simulink model "gm_HDLHeaderScrambler_vs"  (R2024a)
settings: Solver=FixedStepDiscrete  StartTime=0.0  StopTime=stopTime  RelTol=1e-3
values from neighbouring files (symbols this model uses):
  fs = 1    [testHeaderScrambler.m]
undefined symbols (not defined in the file or in its folder): clk, clk_enable, reset_x
libraries: hdlsllib x23, simulink x4, dspsrcs4 x2, whdlutilities x1, vivadosimlib x1, HDL_ieee_8021513 x1
settings Model: Creator=cotti  LastModifiedBy=cotti
settings OptimizationCC: BlockReduction=off  ConditionallyExecuteInputs=off  DefaultParameterBehavior=Inlined  InheritOutputTypeSmallerThanSingle=on
settings DebuggingCC: AlgebraicLoopMsg=error  ArtificialAlgebraicLoopMsg=error  InheritedTsInSrcMsg=none  SingleTaskRateTransMsg=error  UnconnectedInputMsg=warning  UnconnectedOutputMsg=warning  UnconnectedLineMsg=warning
settings HardwareCC: ProdBitPerPointer=32  ProdBitPerSizeT=32  ProdBitPerPtrDiffT=32  ProdLargestAtomicFloat=None  ProdIntDivRoundTo=Undefined  ProdEndianess=Unspecified  ProdWordSize=32  ProdHWDeviceType=ASIC/FPGA->ASIC/FPGA  TargetBitPerLong=64  TargetBitPerPointer=64  TargetBitPerSizeT=64  TargetBitPerPtrDiffT=64  TargetLongLongMode=on  TargetIntDivRoundTo=Zero  TargetEndianess=LittleEndian  TargetWordSize=64  TargetHWDeviceType=Custom Processor->MATLAB Host Computer  ProdEqTarget=off

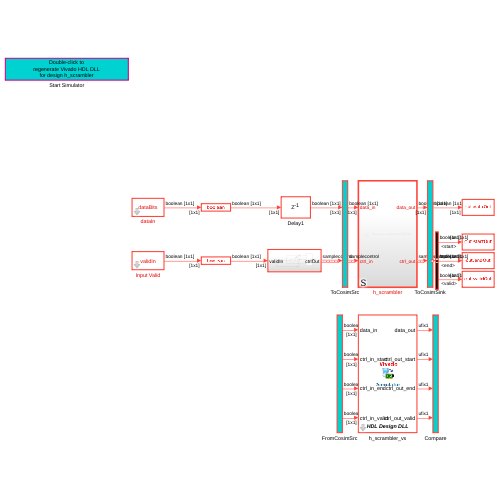
[thumbnail: Simulink's stored preview of the top-level diagram]
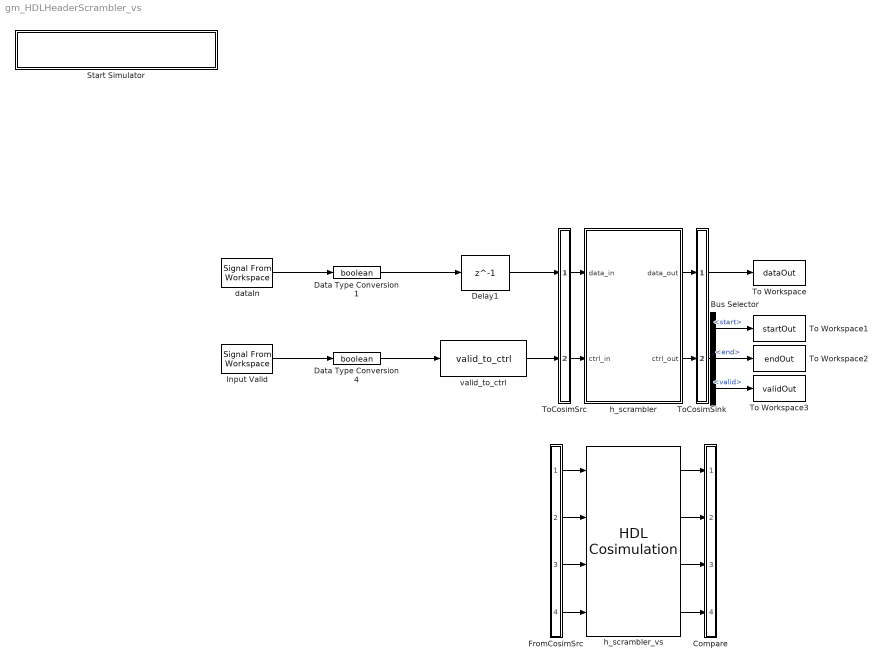
== system gm_HDLHeaderScrambler_vs ==
  Bus Selector : BusSelector  OutputSignals=start,end,valid
  Compare : Subsystem
      mask Display: disp('')
  Data Type Conversion1 : DataTypeConversion  OutDataTypeStr=boolean  SaturateOnIntegerOverflow=off  RndMeth=Floor
  Data Type Conversion4 : DataTypeConversion  OutDataTypeStr=boolean  SaturateOnIntegerOverflow=off  RndMeth=Floor
  Delay1 : Delay  DelayLength=1  InitialCondition=0  UseCircularBuffer=on
  FromCosimSrc : Subsystem
      mask Display: disp('')
  Input Valid : dspsrcs4/Signal From Workspace  X=validIn  Ts=1/fs  nsamps=1  OutputAfterFinalValue=Setting to zero  ignoreOrWarnInputAndFrameLengths=off  OutputFrames=off
  Start Simulator : Subsystem
      settings: OpenFcn=|
      | cosimDirName = pwd;
      | cd 'hdl_prj/hdlsrc/HDLHeaderScrambler';
      | [s,r] = system('vivado -mode batch -source gm_HDLHeaderScrambler_vs.tcl','-echo');
      | cd (cosimDirName);
      | clear cosimDirName;
      | if s
      |    error('Failed to create Vivado HDL design DLL using script gm_HDLHeaderScrambler_vs.tcl.');
      | end
      mask Display: disp('Double-click to\nregenerate Vivado HDL DLL\nfor design h_scrambler')
  To Workspace : ToWorkspace  VariableName=dataOut  SampleTime=1/fs
      settings: Save2DSignal=2-D array (concatenate along first dimension)
  To Workspace1 : ToWorkspace  VariableName=startOut  SampleTime=1/fs
      settings: Save2DSignal=2-D array (concatenate along first dimension)
  To Workspace2 : ToWorkspace  VariableName=endOut  SampleTime=1/fs
      settings: Save2DSignal=2-D array (concatenate along first dimension)
  To Workspace3 : ToWorkspace  VariableName=validOut  SampleTime=1/fs
      settings: Save2DSignal=2-D array (concatenate along first dimension)
  ToCosimSink : Subsystem
      mask Display: disp('')
  ToCosimSrc : Subsystem
      mask Display: disp('')
  dataIn : dspsrcs4/Signal From Workspace  X=dataBits  Ts=1/fs  nsamps=1  OutputAfterFinalValue=Setting to zero  ignoreOrWarnInputAndFrameLengths=off  OutputFrames=off
  h_scrambler : Subsystem
      settings: LibrarySourceBlock=|
      | hdlsllib/Ports &
      | Subsystems/Subsystem
  h_scrambler_vs : vivadosimlib/HDL Cosimulation  PortPaths=/h_scrambler/data_in;/h_scrambler/ctrl_in_start;/h_scrambler/ctrl_in_end;/h_scrambler/ctrl_in_valid;/h_scrambler/data_out;/h_scrambler/ctrl_out_start;/h_scrambler/ctrl_out_end;/h_scrambler/ctrl_out_valid  PortModes=[1 1 1 1 2 2 2 2 ]  PortTimes=[-1 -1 -1 -1 1 1 1 1 ]  PortSigns=[-1 -1 -1 -1 0 0 0 0 ]  PortFracLengths=[0,0,0,0,0,0,0,0]  PortWordLengths=[-1,-1,-1,-1,1,1,1,1]  PortHDLWordSizes=[1,1,1,1,1,1,1,1]  CommLocal=on  CommSharedMemory=on  CommPortNumber=4449  CommShowInfo=on  ClockPaths=clk;clk_enable;reset_x;  ClockModes=[2 4 3]  ClockTimes=[1e-08 3.7e-08 2.7e-08]  TclPostSimCommand="puts \"done\""  TimingMode=ns  TimingScaleFactor=10  idxCellArray={'UNUSED_VAR'}  CosimBypass=Full Simulation  AllowDirectFeedthrough=on  ProductName=EDA Simulator Link VS  RunAutoTimescale=off  HdlClocks=0  PreRunTime=40  PreRunTimeUnit=ns
  valid_to_ctrl : HDL_ieee_8021513/valid_to_ctrl  SystemSampleTime=-1  VariantActivationTime=update diagram  AllowFlexibleInterface=on  Latency=0  AutoFrameSizeCalculation=off
      settings: SourceProductName=HDL IEEE 8021513
  wires:
  Bus Selector/2 -> To Workspace2/1  "<end>"
  Bus Selector/3 -> To Workspace3/1  "<valid>"
  Bus Selector/1 -> To Workspace1/1  "<start>"
  Data Type Conversion1/1 -> Delay1/1
  dataIn/1 -> Data Type Conversion1/1
  Data Type Conversion4/1 -> valid_to_ctrl/1
  Input Valid/1 -> Data Type Conversion4/1
  ToCosimSrc/1(out1) -> h_scrambler/1(data_in)
  ToCosimSrc/2(out2) -> h_scrambler/2(ctrl_in)
  h_scrambler/1(data_out) -> ToCosimSink/1(in1)
  h_scrambler/2(ctrl_out) -> ToCosimSink/2(in2)
  Delay1/1 -> ToCosimSrc/1(in1)
  valid_to_ctrl/1 -> ToCosimSrc/2(in2)
  ToCosimSink/1(out1) -> To Workspace/1
  ToCosimSink/2(out2) -> Bus Selector/1
  FromCosimSrc/1(out1) -> h_scrambler_vs/1
  FromCosimSrc/2(out2) -> h_scrambler_vs/2
  FromCosimSrc/3(out3) -> h_scrambler_vs/3
  FromCosimSrc/4(out4) -> h_scrambler_vs/4
  h_scrambler_vs/1 -> Compare/1(in1)
  h_scrambler_vs/2 -> Compare/2(in2)
  h_scrambler_vs/3 -> Compare/3(in3)
  h_scrambler_vs/4 -> Compare/4(in4)

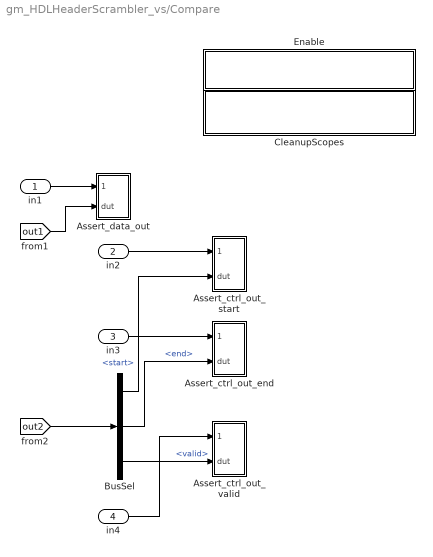
== system gm_HDLHeaderScrambler_vs/Compare ==
  in1 : Inport
  in2 : Inport  Port=2
  in3 : Inport  Port=3
  in4 : Inport  Port=4
  Assert_ctrl_out_end : Subsystem
      settings: LibrarySourceBlock=hdlmdlgenlib/AssertEq
  Assert_ctrl_out_start : Subsystem
      settings: LibrarySourceBlock=hdlmdlgenlib/AssertEq
  Assert_ctrl_out_valid : Subsystem
      settings: LibrarySourceBlock=hdlmdlgenlib/AssertEq
  Assert_data_out : Subsystem
      settings: LibrarySourceBlock=hdlmdlgenlib/AssertEq
  BusSel : BusSelector  OutputSignals=start,end,valid
  CleanupScopes : Subsystem
      settings: OpenFcn=|
      | blkName = gcb; %self block
      | idx = regexp(blkName, '/CleanupScopes$', 'once');
      | blkParent = blkName(1:idx-1);
      | blks=find_system(blkParent, 'LookUnderMasks', 'all','blocktype', 'Scope');
      | for itr = 1:length(blks)
      | 	 hScopeCfg = get_param(blks{itr},'ScopeConfiguration');
      | 	 hScopeCfg.Visible = ~ hScopeCfg.Visible;
      | end
      | drawnow;
      mask Display: fprintf(message('hdlcoder:cosim:vnl_dblclick').getString());
  Enable : Subsystem
      settings: OpenFcn=|
      | blkName = gcb;
      | idx = regexp(blkName, '/Enable$', 'once');
      | blkParent = blkName(1:idx-1);
      | blks=find_system(blkParent, 'LookUnderMasks', 'all','blocktype', 'Assertion');
      | e = get_param(blks{1}, 'Enabled');
      | if strcmp(e, 'on'), f= 'off';, else, f = 'on';, end
      | for ii=1:length(blks), set_param(blks{ii}, 'Enabled', f);, end
      | set_param(gcb, 'MaskDisplay',['fprintf(message(''hdlcoder:cosim:vnl_dblclick_assertions'',','''',upper(e),'''',').getString())']);
      mask Display: fprintf(message('hdlcoder:cosim:vnl_dblclick_assertions','OFF').getString());
  wires:
  BusSel/1 -> Assert_ctrl_out_start/2(dut)  "<start>"
  BusSel/3 -> Assert_ctrl_out_valid/2(dut)  "<valid>"
  BusSel/2 -> Assert_ctrl_out_end/2(dut)  "<end>"
  in3/1 -> Assert_ctrl_out_end/1(cosim)
  in2/1 -> Assert_ctrl_out_start/1(cosim)
  in4/1 -> Assert_ctrl_out_valid/1(cosim)
  [out2] -> BusSel/1
  [out1] -> Assert_data_out/2(dut)
  in1/1 -> Assert_data_out/1(cosim)

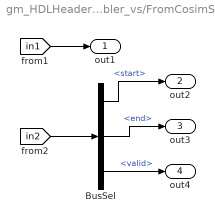
== system gm_HDLHeaderScrambler_vs/FromCosimSrc ==
  BusSel : BusSelector  OutputSignals=start,end,valid
  out1 : Outport
  out2 : Outport  Port=2
  out3 : Outport  Port=3
  out4 : Outport  Port=4
  wires:
  BusSel/3 -> out4/1  "<valid>"
  BusSel/2 -> out3/1  "<end>"
  BusSel/1 -> out2/1  "<start>"
  [in2] -> BusSel/1
  [in1] -> out1/1

== system gm_HDLHeaderScrambler_vs/Start Simulator ==

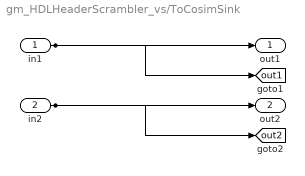
== system gm_HDLHeaderScrambler_vs/ToCosimSink ==
  in1 : Inport
  in2 : Inport  Port=2
  out1 : Outport
  out2 : Outport  Port=2
  tag scope: out1=global, out2=global
  wires:
  in1/1 -> out1/1, [out1]
  in2/1 -> out2/1, [out2]

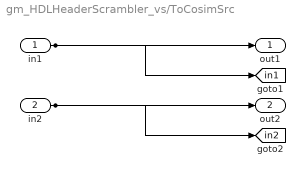
== system gm_HDLHeaderScrambler_vs/ToCosimSrc ==
  in1 : Inport
  in2 : Inport  Port=2
  out1 : Outport
  out2 : Outport  Port=2
  tag scope: in1=global, in2=global
  wires:
  in1/1 -> out1/1, [in1]
  in2/1 -> out2/1, [in2]

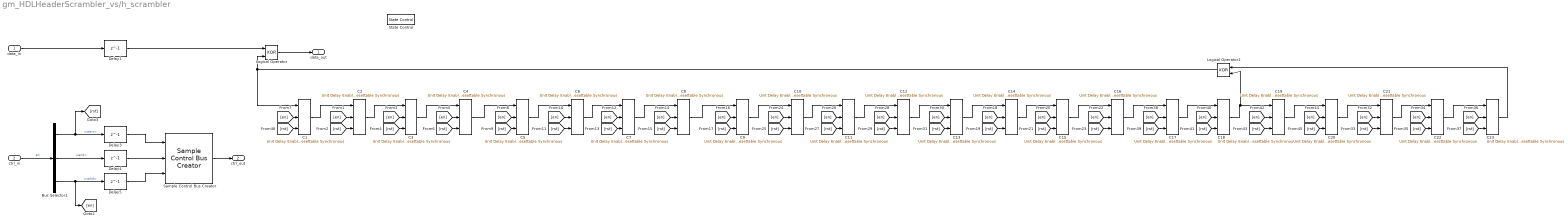
== system gm_HDLHeaderScrambler_vs/h_scrambler ==
  data_in : Inport
  ctrl_in : Inport  Port=2
  Bus Selector1 : BusSelector  OutputSignals=start,end,valid
  C{1,3,5,7,9,11,13,15,17,19,21,23} (12 alike) : hdlsllib/Discrete/Unit Delay Enabled Resettable Synchronous  InitialCondition=0  SampleTime=-1
  C{2,4,6,8,10,12,14,16,18,20,22} (11 alike) : hdlsllib/Discrete/Unit Delay Enabled Resettable Synchronous  InitialCondition=1  SampleTime=-1
  Delay{1,3..5} (4 alike) : Delay  DelayLength=1  InitialCondition=0  UseCircularBuffer=on
  Logical Operator : Logic  Operator=XOR  IconShape=distinctive  AllPortsSameDT=off  OutDataTypeStr=boolean
  Logical Operator1 : Logic  Operator=XOR  IconShape=distinctive  AllPortsSameDT=off  OutDataTypeStr=boolean
  Sample Control Bus Creator : whdlutilities/Sample Control Bus Creator
  State Control : StateControl  StateControl=Synchronous
  data_out : Outport
  ctrl_out : Outport  Port=2  VectorParamsAs1DForOutWhenUnconnected=off
  wires:
  Sample Control Bus Creator/1 -> ctrl_out/1
  Delay5/1 -> Sample Control Bus Creator/3
  Delay4/1 -> Sample Control Bus Creator/2
  Delay3/1 -> Sample Control Bus Creator/1
  Bus Selector1/3 -> Delay5/1, [en]  "<valid>"
  Bus Selector1/2 -> Delay4/1  "<end>"
  Bus Selector1/1 -> Delay3/1, [rst]  "<start>"
  C23/1 -> Logical Operator1/1
  [rst] -> C22/3
  C19/1 -> C20/1
  [en] -> C20/2
  [en] -> C21/2
  C21/1 -> C22/1
  [rst] -> C18/3
  [en] -> C17/2
  [rst] -> C19/3
  [rst] -> C21/3
  C17/1 -> C18/1
  C22/1 -> C23/1
  [en] -> C19/2
  [en] -> C18/2
  [en] -> C23/2
  [rst] -> C20/3
  [en] -> C22/2
  C16/1 -> C17/1
  [rst] -> C23/3
  [rst] -> C17/3
  C8/1 -> C9/1
  [rst] -> C15/3
  [en] -> C15/2
  [en] -> C14/2
  [rst] -> C16/3
  [en] -> C12/2
  [rst] -> C14/3
  C13/1 -> C14/1
  C11/1 -> C12/1
  [rst] -> C9/3
  [en] -> C10/2
  [en] -> C9/2
  C14/1 -> C15/1
  [en] -> C11/2
  [rst] -> C13/3
  C10/1 -> C11/1
  [rst] -> C10/3
  C12/1 -> C13/1
  [en] -> C13/2
  [rst] -> C11/3
  [en] -> C16/2
  [rst] -> C12/3
  C9/1 -> C10/1
  C15/1 -> C16/1
  [rst] -> C5/3
  [en] -> C6/2
  C6/1 -> C7/1
  [en] -> C8/2
  [rst] -> C6/3
  C5/1 -> C6/1
  [rst] -> C7/3
  C7/1 -> C8/1
  [rst] -> C8/3
  [en] -> C7/2
  [en] -> C5/2
  Delay1/1 -> Logical Operator/1
  data_in/1 -> Delay1/1
  ctrl_in/1 -> Bus Selector1/1  "en"
  Logical Operator/1 -> data_out/1
  [rst] -> C3/3
  [en] -> C3/2
  Logical Operator1/1 -> Logical Operator/2, C1/1
  [rst] -> C2/3
  C1/1 -> C2/1
  C3/1 -> C4/1
  [en] -> C1/2
  [rst] -> C1/3
  C4/1 -> C5/1
  [en] -> C4/2
  C2/1 -> C3/1
  [rst] -> C4/3
  [en] -> C2/2
  C20/1 -> C21/1
  C18/1 -> Logical Operator1/2, C19/1

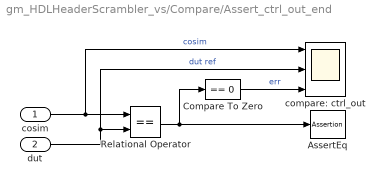
== system gm_HDLHeaderScrambler_vs/Compare/Assert_ctrl_out_end ==
  cosim : Inport
  dut : Inport  Port=2
  AssertEq : Assertion
  Compare To Zero : simulink/Logic and Bit Operations/Compare To Zero  relop===  OutDataTypeStr=boolean
  Relational Operator : RelationalOperator  Operator===  OutDataTypeStr=boolean  InputSameDT=off
  compare: ctrl_out : Scope  NumInputPorts=3
  wires:
  Compare To Zero/1 -> compare: ctrl_out/3  "err"
  Relational Operator/1 -> Compare To Zero/1, AssertEq/1
  cosim/1 -> compare: ctrl_out/1, Relational Operator/1  "cosim"
  dut/1 -> compare: ctrl_out/2, Relational Operator/2  "dut ref"

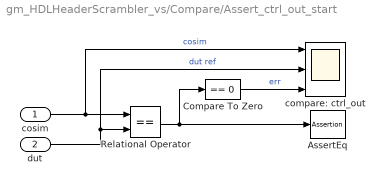
== system gm_HDLHeaderScrambler_vs/Compare/Assert_ctrl_out_start ==
  cosim : Inport
  dut : Inport  Port=2
  AssertEq : Assertion
  Compare To Zero : simulink/Logic and Bit Operations/Compare To Zero  relop===  OutDataTypeStr=boolean
  Relational Operator : RelationalOperator  Operator===  OutDataTypeStr=boolean  InputSameDT=off
  compare: ctrl_out : Scope  NumInputPorts=3
  wires:
  Compare To Zero/1 -> compare: ctrl_out/3  "err"
  Relational Operator/1 -> Compare To Zero/1, AssertEq/1
  cosim/1 -> compare: ctrl_out/1, Relational Operator/1  "cosim"
  dut/1 -> compare: ctrl_out/2, Relational Operator/2  "dut ref"

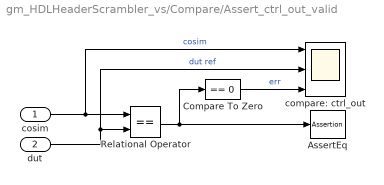
== system gm_HDLHeaderScrambler_vs/Compare/Assert_ctrl_out_valid ==
  cosim : Inport
  dut : Inport  Port=2
  AssertEq : Assertion
  Compare To Zero : simulink/Logic and Bit Operations/Compare To Zero  relop===  OutDataTypeStr=boolean
  Relational Operator : RelationalOperator  Operator===  OutDataTypeStr=boolean  InputSameDT=off
  compare: ctrl_out : Scope  NumInputPorts=3
  wires:
  Compare To Zero/1 -> compare: ctrl_out/3  "err"
  Relational Operator/1 -> Compare To Zero/1, AssertEq/1
  cosim/1 -> compare: ctrl_out/1, Relational Operator/1  "cosim"
  dut/1 -> compare: ctrl_out/2, Relational Operator/2  "dut ref"

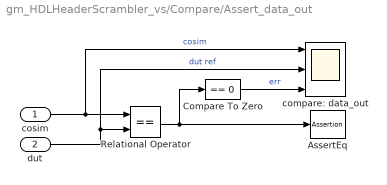
== system gm_HDLHeaderScrambler_vs/Compare/Assert_data_out ==
  cosim : Inport
  dut : Inport  Port=2
  AssertEq : Assertion
  Compare To Zero : simulink/Logic and Bit Operations/Compare To Zero  relop===  OutDataTypeStr=boolean
  Relational Operator : RelationalOperator  Operator===  OutDataTypeStr=boolean  InputSameDT=off
  compare: data_out : Scope  NumInputPorts=3
  wires:
  Compare To Zero/1 -> compare: data_out/3  "err"
  Relational Operator/1 -> Compare To Zero/1, AssertEq/1
  cosim/1 -> compare: data_out/1, Relational Operator/1  "cosim"
  dut/1 -> compare: data_out/2, Relational Operator/2  "dut ref"

== system gm_HDLHeaderScrambler_vs/Compare/CleanupScopes ==

== system gm_HDLHeaderScrambler_vs/Compare/Enable ==
